simulink model "Control_Gain"  (R2021a)
settings: Solver=VariableStepAuto  StartTime=0.0  StopTime=10.0  RelTol=1e-3
settings Model: Creator=my computer  LastModifiedBy=my computer

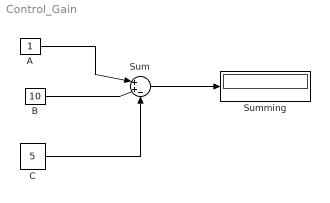
== system Control_Gain ==
  A : Constant
  B : Constant  Value=10
  C : Constant  Value=5
  Sum : Sum  Inputs=|++-
  Summing : Display
  wires:
  A/1 -> Sum/1
  B/1 -> Sum/2
  Sum/1 -> Summing/1
  C/1 -> Sum/3
